simulink model "Power"  (R2015b)
settings: Solver=VariableStepAuto  StartTime=0.0  StopTime=0  RelTol=1e-3
libraries: commdigbbndpm3 x5, commrandsrc3 x2, commsink2 x2
settings Model: Creator=Lucifer  LastModifiedBy=Lucifer

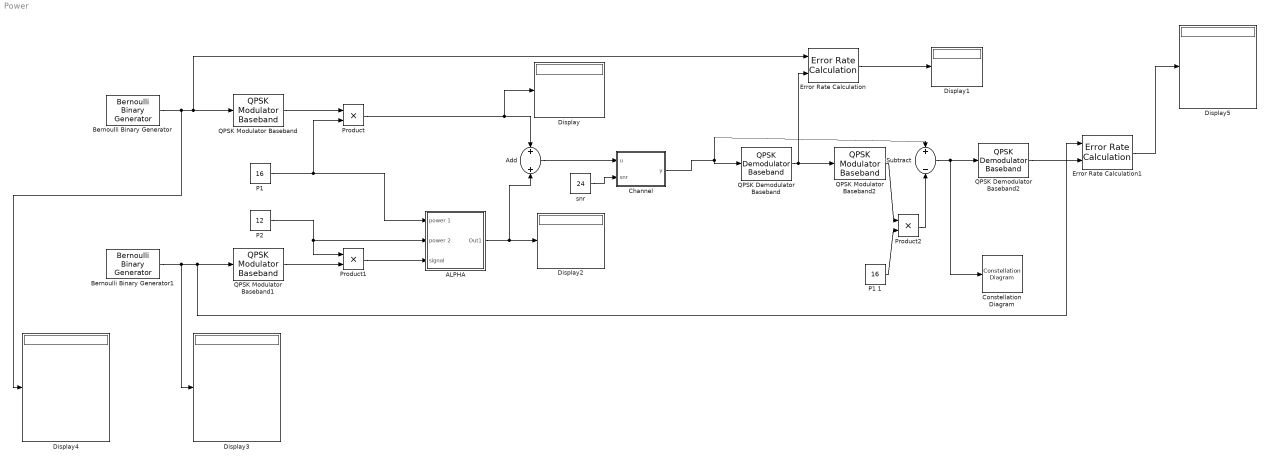
== system Power ==
  "ALPHA " : Subsystem
  Add : Sum
  Bernoulli Binary Generator : commrandsrc3/Bernoulli Binary Generator  ProbabilityOfZero=0.5  SeedSource=Auto  Seed=0  SampleTime=1  SamplesPerFrame=100000  OutputDataType=double  SimulateUsing=Interpreted execution
  Bernoulli Binary Generator1 : commrandsrc3/Bernoulli Binary Generator  ProbabilityOfZero=0.5  SeedSource=Auto  Seed=0  SampleTime=1  SamplesPerFrame=100000  OutputDataType=double  SimulateUsing=Interpreted execution
  "Channel " : MATLAB Function  TreatAsAtomicUnit=on
  Constellation Diagram : ConstellationDiagram
  Display{,1..5} (6 alike) : Display
  Error Rate Calculation : commsink2/Error Rate Calculation  N=0  st_delay=0  cp_mode=Entire frame  subframe=[]  PMode=Port  WsName=ErrorVec  RsMode2=off  stop=off  numErr=100  maxBits=1e6
  Error Rate Calculation1 : commsink2/Error Rate Calculation  N=0  st_delay=0  cp_mode=Entire frame  subframe=[]  PMode=Port  WsName=ErrorVec  RsMode2=off  stop=off  numErr=100  maxBits=1e6
  "P1 " : Constant  Value=16
  P1 1 : Constant  Value=16
  P2 : Constant  Value=12
  Product : Product
  Product1 : Product
  Product2 : Product
  QPSK Demodulator Baseband : commdigbbndpm3/QPSK Demodulator Baseband  Ph=pi/4  Dec=Binary  OutType=Bit  DecType=Hard decision  VarSource=Dialog  Variance=1  outDtype1=Inherit via internal rule  outDtype2=Inherit via internal rule  derotateFactorWordLen=16
  QPSK Demodulator Baseband2 : commdigbbndpm3/QPSK Demodulator Baseband  Ph=pi/4  Dec=Binary  OutType=Bit  DecType=Hard decision  VarSource=Dialog  Variance=1  outDtype1=Inherit via internal rule  outDtype2=Inherit via internal rule  derotateFactorWordLen=16
  QPSK Modulator Baseband : commdigbbndpm3/QPSK Modulator Baseband  InType=Bit  Enc=Binary  Ph=pi/4  outDtype=double  outWordLen=16  outUDDataType=sfix(16)  outFracLenMode=Best precision  outFracLen=15
  QPSK Modulator Baseband1 : commdigbbndpm3/QPSK Modulator Baseband  InType=Bit  Enc=Binary  Ph=pi/4  outDtype=double  outWordLen=16  outUDDataType=sfix(16)  outFracLenMode=Best precision  outFracLen=15
  QPSK Modulator Baseband2 : commdigbbndpm3/QPSK Modulator Baseband  InType=Bit  Enc=Binary  Ph=pi/4  outDtype=double  outWordLen=16  outUDDataType=sfix(16)  outFracLenMode=Best precision  outFracLen=15
  Subtract : Sum  Inputs=+-
  "snr " : Constant  Value=24
  wires:
  Bernoulli Binary Generator/1 -> Display4/1, Error Rate Calculation/1, QPSK Modulator Baseband/1
  QPSK Modulator Baseband/1 -> Product/1
  "P1 "/1 -> Product/2, "ALPHA "/1(power 1)
  QPSK Modulator Baseband1/1 -> Product1/2
  P2/1 -> "ALPHA "/2(power 2), Product1/1
  Product/1 -> Display/1, Add/1
  QPSK Demodulator Baseband/1 -> Error Rate Calculation/2, QPSK Modulator Baseband2/1
  Error Rate Calculation/1 -> Display1/1
  Error Rate Calculation1/1 -> Display5/1
  QPSK Demodulator Baseband2/1 -> Error Rate Calculation1/2
  Product1/1 -> "ALPHA "/3(signal)
  "ALPHA "/1(Out1) -> Add/2, Display2/1
  Bernoulli Binary Generator1/1 -> Display3/1, Error Rate Calculation1/1, QPSK Modulator Baseband1/1
  P1 1/1 -> Product2/2
  QPSK Modulator Baseband2/1 -> Product2/1
  Product2/1 -> Subtract/2
  Add/1 -> "Channel "/1(u)
  "Channel "/1(y) -> QPSK Demodulator Baseband/1, Subtract/1
  "snr "/1 -> "Channel "/2(snr)
  Subtract/1 -> Constellation Diagram/1, QPSK Demodulator Baseband2/1

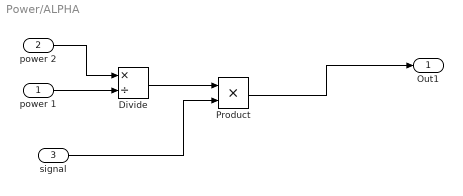
== system Power/ALPHA  ==
  power 1 : Inport
  power 2 : Inport  Port=2
  signal : Inport  Port=3
  Divide : Product  Inputs=*/
  Product : Product
  Out1 : Outport
  wires:
  power 2/1 -> Divide/1
  power 1/1 -> Divide/2
  Divide/1 -> Product/1
  signal/1 -> Product/2
  Product/1 -> Out1/1

== matlab function Power/Channel  ==
  data: u input; y output; snr input
function y = fcn(u,snr)

n=length(u);
y=zeros(n,1)+1j*zeros(n,1);
h= rand(n,1) + 1j*rand(n,1);
noise = rand(n,1) + 1j*rand(n,1);
n_var = 10^(-snr/20);
y=(h.*u)+(noise)*sqrt(n_var);    
y=y./h;
end
